simulink model "MagicFormulaloadingvariables"  (R2024b)
settings: Solver=VariableStepAuto  StartTime=0.0  StopTime=30  RelTol=1e-3
undefined symbols (not defined in the file or in its folder): PCY1, PDY1, PDY2, PDY3, PEY1, PEY2, PEY3, PEY4, PHY1, PHY2, PKY1, PKY2, PKY3, PVY1, PVY2, PVY3, PVY4
libraries: simulink x1
settings Model: Creator=rober  LastModifiedBy=rober

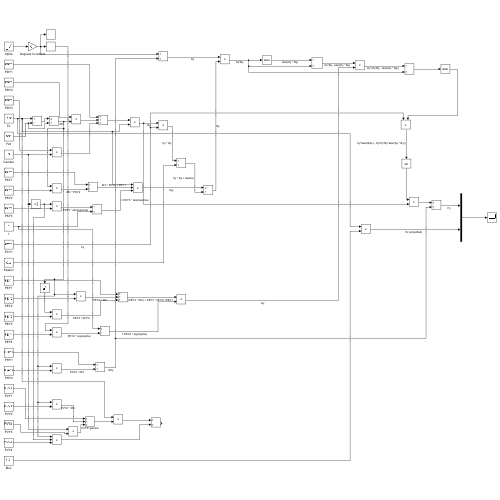
[thumbnail: Simulink's stored preview of the top-level diagram]
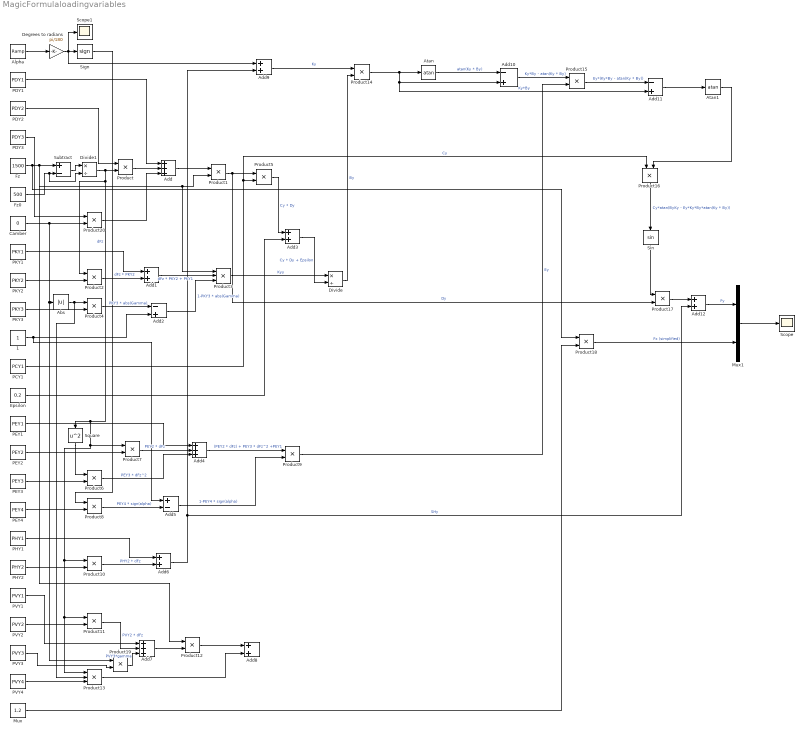
== system MagicFormulaloadingvariables ==
  1 : Constant
  Abs : Abs  SaturateOnIntegerOverflow=off
  Add : Sum  Inputs=+++
  Add{1,3,6,8..9,12} (6 alike) : Sum
  Add10 : Sum  Inputs=-+
  Add11 : Sum  Inputs=-+
  Add2 : Sum  Inputs=-+
  Add4 : Sum  Inputs=+++
  Add5 : Sum  Inputs=+-
  Add7 : Sum  Inputs=+++
  Alpha : simulink/Sources/Ramp  slope=1  start=0  InitialOutput=-15
  Atan : Trigonometry  Operator=atan
  Atan1 : Trigonometry  Operator=atan
  Camber : Constant  Value=0
  Degrees to radians : Gain  Gain=pi/180
  Divide : Product  Inputs=*/
  Divide1 : Product  Inputs=*/
  Epsilon : Constant  Value=0.2
  Fz : Constant  Value=1500
  Fz0 : Constant  Value=500
  Mux : Constant  Value=1.2
  Mux1 : Mux  Inputs=2
  PCY1 : Constant  Value=PCY1
  PDY1 : Constant  Value=PDY1
  PDY2 : Constant  Value=PDY2
  PDY3 : Constant  Value=PDY3
  PEY1 : Constant  Value=PEY1
  PEY2 : Constant  Value=PEY2
  PEY3 : Constant  Value=PEY3
  PEY4 : Constant  Value=PEY4
  PHY1 : Constant  Value=PHY1
  PHY2 : Constant  Value=PHY2
  PKY1 : Constant  Value=PKY1
  PKY2 : Constant  Value=PKY2
  PKY3 : Constant  Value=PKY3
  PVY1 : Constant  Value=PVY1
  PVY2 : Constant  Value=PVY2
  PVY3 : Constant  Value=PVY3
  PVY4 : Constant  Value=PVY4
  Product{,1..2,4..12,14..20} (19 alike) : Product
  Product13 : Product  Inputs=3
  Product3 : Product  Inputs=3
  Scope : Scope
  Scope1 : Scope
  Sign : Signum
  Sin : Trigonometry
  Square : Math  Operator=square
  Subtract : Sum  Inputs=+-
  wires:
  Fz/1 -> Product18/1, Product12/1, Product3/1, Product1/2, Subtract/1
  Fz0/1 -> Divide1/2, Subtract/2
  Subtract/1 -> Divide1/1
  PDY2/1 -> Product/1
  Camber/1 -> Product20/2, Product19/1, Abs/1
  PDY3/1 -> Product20/1
  Product/1 -> Add/2
  Product20/1 -> Add/3
  PDY1/1 -> Add/1
  Add/1 -> Product1/1
  Product1/1 -> Product17/2, Product5/1  "Dy"
  PKY2/1 -> Product2/2
  Product2/1 -> Add1/2  "dFz * PKY2"
  PKY1/1 -> Add1/1
  Add1/1 -> Product3/2  "dFz * PKY2 + PKY1"
  PKY3/1 -> Product4/2
  Product4/1 -> Add2/1  "PKY3 * abs(Gamma)"
  Abs/1 -> Product13/2, Product4/1
  1/1 -> Add5/1, Add2/2
  Add2/1 -> Product3/3  "1-PKY3 * abs(Gamma)"
  Product3/1 -> Divide/1  "Kyy"
  PCY1/1 -> Product16/1, Product5/2  "Cy"
  Product5/1 -> Add3/1  "Cy * Dy"
  Epsilon/1 -> Add3/2
  Add3/1 -> Divide/2  "Cy * Dy + Epsilon"
  Divide/1 -> Product14/2  "By"
  PEY3/1 -> Product6/2
  Square/1 -> Product6/1
  PEY2/1 -> Product7/2
  Product7/1 -> Add4/2  "PEY2 * dFz"
  Product6/1 -> Add4/3  "PEY3 * dFz^2"
  PEY1/1 -> Add4/1
  Alpha/1 -> Degrees to radians/1
  PEY4/1 -> Product8/2
  Sign/1 -> Product8/1
  Product8/1 -> Add5/2  "PEY4 * sign(alpha)"
  Add5/1 -> Product9/2  "1-PEY4 * sign(alpha)"
  Add4/1 -> Product9/1  "(PEY2 * dFz) + PEY3 * dFz^2 +PEY1"
  Product9/1 -> Product15/2  "Ey"
  PHY2/1 -> Product10/2
  Divide1/1 -> Product2/1, Product13/1, Product11/1, Product10/1, Product7/1, Square/1, Product/2  "dFz"
  Product10/1 -> Add6/2  "PHY2 * dFz"
  PHY1/1 -> Add6/1
  PVY2/1 -> Product11/2
  PVY1/1 -> Add7/1
  Product11/1 -> Add7/2  "PVY2 * dFz"
  Add7/1 -> Product12/2
  Product12/1 -> Add8/1
  PVY4/1 -> Product13/3
  Product13/1 -> Add8/2
  Add6/1 -> Add12/2, Add9/2  "SHy"
  Add9/1 -> Product14/1  "Ky"
  Product14/1 -> Add11/2, Add10/2, Atan/1  "Ky*By"
  Atan/1 -> Add10/1  "atan(Ky * By)"
  Add10/1 -> Product15/1  "Ky*By - atan(Ky * By)"
  Product15/1 -> Add11/1  "Ey*(Ky*By - atan(Ky * By))"
  Add11/1 -> Atan1/1
  Atan1/1 -> Product16/2
  Product16/1 -> Sin/1  "Cy*atan(ByKy - Ey*Ky*By*atan(Ky * By))"
  Sin/1 -> Product17/1
  Mux/1 -> Product18/2
  Product18/1 -> Mux1/2  "Fx (simplified)"
  Mux1/1 -> Scope/1
  PVY3/1 -> Product19/2
  Product19/1 -> Add7/3  "PVY3*gamma"
  Product17/1 -> Add12/1
  Add12/1 -> Mux1/1  "Fy"
  Degrees to radians/1 -> Add9/1, Scope1/1, Sign/1
